simulink model "SVPWM2017a"  (R2017a)
settings: Solver=FixedStepAuto  StartTime=0.0  StopTime=0.1  RelTol=1e-3
values from neighbouring files (symbols this model uses):
  pxyz = sqrt(3) *Tsw / Vdc    [setting.m]
  Tsw = 1 / fsw    (= 0.0001)    [setting.m]
  Vdc = 500    [setting.m]
libraries: powerlib x11, simulink x4, powerlib_meascontrol x1
settings Model: Creator=d  LastModifiedBy=d
settings DataIOCC: ReturnWorkspaceOutputs=on
settings DebuggingCC: UnconnectedInputMsg=none  UnconnectedOutputMsg=none  UnconnectedLineMsg=none
settings ModelReferenceCC: EnableRefExpFcnMdlSchedulingChecks=off
settings SFSimCC: SimUseLocalCustomCode=on
settings RTWCC: RTWUseLocalCustomCode=on

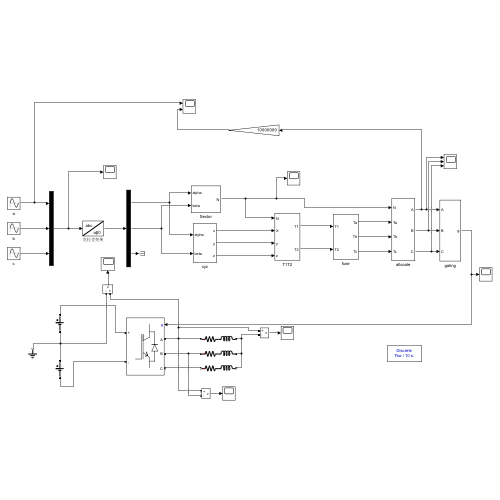
[thumbnail: Simulink's stored preview of the top-level diagram]
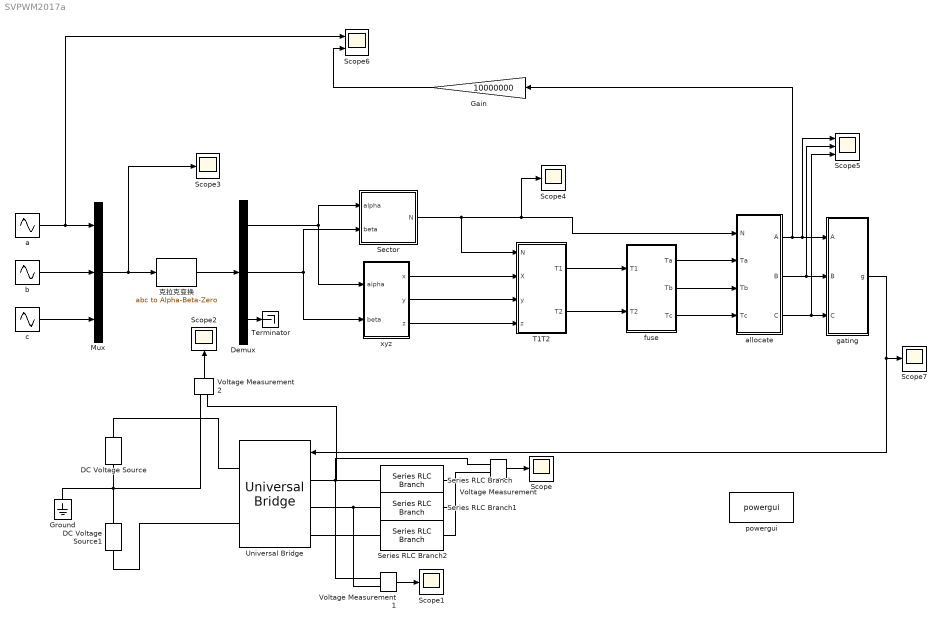
== system SVPWM2017a ==
  DC Voltage Source : powerlib/Electrical Sources/DC Voltage Source  Amplitude=Vdc / 2  Measurements=None
  DC Voltage Source1 : powerlib/Electrical Sources/DC Voltage Source  Amplitude=Vdc / 2  Measurements=None
  Demux : Demux  Outputs=3
  Gain : Gain  Gain=10000000
  Ground : powerlib/Elements/Ground  LConnTagsString=a
  Mux : Mux  Inputs=3
  Scope{,1..4,7} (6 alike) : Scope
  Scope5 : Scope  NumInputPorts=3
  Scope6 : Scope  NumInputPorts=2
  Sector : Subsystem
  Series RLC Branch : powerlib/Elements/Series RLC Branch  LConnTagsString=__new0  RConnTagsString=__new0  BranchType=RL  Resistance=1  Inductance=1e-3  SetiL0=off  InitialCurrent=0  Capacitance=1e-6  Setx0=off  InitialVoltage=0  Measurements=None
  Series RLC Branch1 : powerlib/Elements/Series RLC Branch  LConnTagsString=__new0  RConnTagsString=__new0  BranchType=RL  Resistance=1  Inductance=1e-3  SetiL0=off  InitialCurrent=0  Capacitance=1e-6  Setx0=off  InitialVoltage=0  Measurements=None
  Series RLC Branch2 : powerlib/Elements/Series RLC Branch  LConnTagsString=__new0  RConnTagsString=__new0  BranchType=RL  Resistance=1  Inductance=1e-3  SetiL0=off  InitialCurrent=0  Capacitance=1e-6  Setx0=off  InitialVoltage=0  Measurements=None
  T1T2 : Subsystem
  Terminator : Terminator
  Universal Bridge : powerlib/Power Electronics/Universal Bridge  Arms=3  SnubberResistance=1e5  SnubberCapacitance=inf  Device=IGBT / Diodes  Ron=1e-3  Lon=0  ForwardVoltages="[  0  0  ]"  ForwardVoltage=0  GTOparameters=[ 10e-6 , 20e-6 ]  IGBTparameters=[ 1e-6 , 2e-6 ]  Measurements=None  Measurements_2=None  converterType=Rectifier
  Voltage Measurement : powerlib/Measurements/Voltage Measurement  PhasorSimulation=off  OutputType=Complex  PSBequivalent=0
  Voltage Measurement1 : powerlib/Measurements/Voltage Measurement  PhasorSimulation=off  OutputType=Complex  PSBequivalent=0
  Voltage Measurement2 : powerlib/Measurements/Voltage Measurement  PhasorSimulation=off  OutputType=Complex  PSBequivalent=0
  a : Sin  Amplitude=(220 * sqrt(2)) / sqrt(3)  Frequency=50*2*pi  SampleTime=0
  allocate : Subsystem
  b : Sin  Amplitude=(220 * sqrt(2)) / sqrt(3)  Frequency=50*2*pi  Phase=-pi*2/3  SampleTime=0
  c : Sin  Amplitude=(220 * sqrt(2)) / sqrt(3)  Frequency=50*2*pi  Phase=-pi*4/3  SampleTime=0
  fuse : Subsystem
  gating : Subsystem
  powergui : powerlib/powergui  Priority=1  SimulationMode=Discrete  SampleTime=Tsw / 10  frequency=60  Iterations=50  frequencyindice=0  Pbase=100e6  ErrMax=1e-4  UnitsV=kV  UnitsW=MW  buscounter=0  FunctionMessages=off  echomessages=off  EnableUseOfTLC=off  CurrentSourceSwitches=off  DisableSnubberDevices=off  DisableRonSwitches=off  DisableVfSwitches=off  DisplayEquations=off  AutomaticDiscreteSolvers=off  SolverType=Tustin/Backward Euler (TBE)  Interpol=off  ExternalGateDelay=off  methode=off  Ts=100  x0status=blocks  SPID=on  SwTol=0  HookPort=off  NonlinearTolerance=1e-4  nMaxIteration=100  ContinueOnMaxIteration=off  RestoreLinks=warning  ResistiveCurrentMeasurement=off  Frange=[0:2:500]  Ylog=off  Xlog=on  ShowGrid=off  save=off  variable=ZData  structure=0  ZoomFFT=off  StartTime=0.0  cycles=1  DisplayStyle=1  fundamental=60  FreqAxis=off  MaxFrequency=1000  frequencyindicesteady=1  RmsSteady=1  display=off
  xyz : Subsystem
  克拉克变换 : powerlib_meascontrol/Transformations/abc to Alpha-Beta-Zero
  wires:
  Sector/1(N) -> T1T2/1(N), Scope4/1, allocate/1(N)
  xyz/1(x) -> T1T2/2(X)
  xyz/2(y) -> T1T2/3(y)
  xyz/3(z) -> T1T2/4(z)
  T1T2/1(T1) -> fuse/1(T1)
  T1T2/2(T2) -> fuse/2(T2)
  fuse/1(Ta) -> allocate/2(Ta)
  fuse/2(Tb) -> allocate/3(Tb)
  fuse/3(Tc) -> allocate/4(Tc)
  allocate/1(A) -> Gain/1, Scope5/1, gating/1(A)
  allocate/2(B) -> Scope5/2, gating/2(B)
  allocate/3(C) -> Scope5/3, gating/3(C)
  a/1 -> Scope6/1, Mux/1
  b/1 -> Mux/2
  c/1 -> Mux/3
  Mux/1 -> Scope3/1, 克拉克变换/1
  克拉克变换/1 -> Demux/1
  Demux/1 -> Sector/1(alpha), xyz/1(alpha)
  Demux/2 -> Sector/2(beta), xyz/2(beta)
  Demux/3 -> Terminator/1
  gating/1(g) -> Scope7/1, Universal Bridge/1
  Voltage Measurement/1 -> Scope/1
  Voltage Measurement1/1 -> Scope1/1
  Voltage Measurement2/1 -> Scope2/1
  Gain/1 -> Scope6/2
  connections:
  DC Voltage Source1/RConn1 -- Voltage Measurement2/LConn2 -- Ground/LConn1 -- DC Voltage Source/LConn1
  DC Voltage Source/RConn1 -- Universal Bridge/RConn1
  DC Voltage Source1/LConn1 -- Universal Bridge/RConn2
  Universal Bridge/LConn1 -- Voltage Measurement2/LConn1 -- Voltage Measurement/LConn1 -- Voltage Measurement1/LConn1 -- Series RLC Branch/LConn1
  Universal Bridge/LConn2 -- Voltage Measurement1/LConn2 -- Series RLC Branch1/LConn1
  Universal Bridge/LConn3 -- Series RLC Branch2/LConn1
  Series RLC Branch/RConn1 -- Voltage Measurement/LConn2 -- Series RLC Branch1/RConn1 -- Series RLC Branch2/RConn1

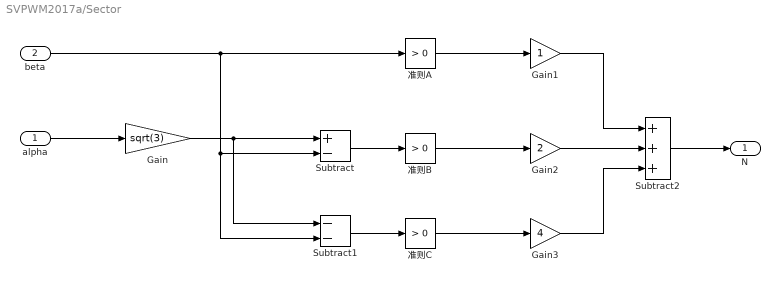
== system SVPWM2017a/Sector ==
  alpha : Inport
  beta : Inport  Port=2
  Gain : Gain  Gain=sqrt(3)
  Gain1 : Gain
  Gain2 : Gain  Gain=2
  Gain3 : Gain  Gain=4
  Subtract : Sum  Inputs=+-
  Subtract1 : Sum  Inputs=--
  Subtract2 : Sum  Inputs=+++
  准则A : simulink/Logic and Bit Operations/Compare To Constant  relop=>  const=0  OutDataTypeStr=boolean
  准则B : simulink/Logic and Bit Operations/Compare To Constant  relop=>  const=0  OutDataTypeStr=boolean
  准则C : simulink/Logic and Bit Operations/Compare To Constant  relop=>  const=0  OutDataTypeStr=boolean
  N : Outport
  wires:
  beta/1 -> Subtract1/2, Subtract/2, 准则A/1
  alpha/1 -> Gain/1
  Gain/1 -> Subtract1/1, Subtract/1
  Subtract/1 -> 准则B/1
  Subtract1/1 -> 准则C/1
  准则C/1 -> Gain3/1
  准则B/1 -> Gain2/1
  准则A/1 -> Gain1/1
  Gain1/1 -> Subtract2/1
  Gain2/1 -> Subtract2/2
  Gain3/1 -> Subtract2/3
  Subtract2/1 -> N/1

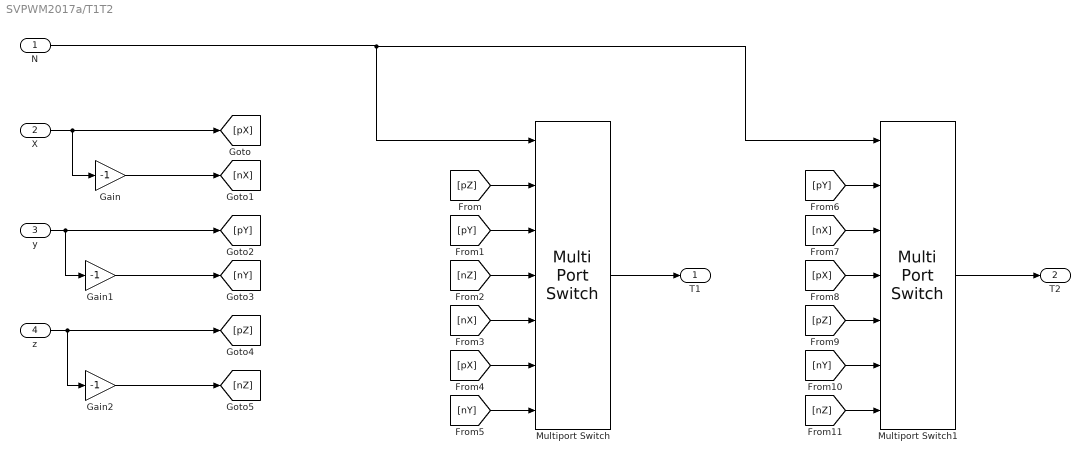
== system SVPWM2017a/T1T2 ==
  N : Inport
  X : Inport  Port=2
  y : Inport  Port=3
  z : Inport  Port=4
  Gain : Gain  Gain=-1
  Gain1 : Gain  Gain=-1
  Gain2 : Gain  Gain=-1
  Multiport Switch : MultiPortSwitch  Inputs=6
  Multiport Switch1 : MultiPortSwitch  Inputs=6
  T1 : Outport
  T2 : Outport  Port=2
  wires:
  X/1 -> [pX], Gain/1
  y/1 -> [pY], Gain1/1
  z/1 -> Gain2/1, [pZ]
  Gain/1 -> [nX]
  Gain1/1 -> [nY]
  Gain2/1 -> [nZ]
  Multiport Switch/1 -> T1/1
  Multiport Switch1/1 -> T2/1
  N/1 -> Multiport Switch1/1, Multiport Switch/1
  [pZ] -> Multiport Switch/2
  [pY] -> Multiport Switch/3
  [nZ] -> Multiport Switch/4
  [nX] -> Multiport Switch/5
  [pX] -> Multiport Switch/6
  [nY] -> Multiport Switch/7
  [pY] -> Multiport Switch1/2
  [nX] -> Multiport Switch1/3
  [pX] -> Multiport Switch1/4
  [pZ] -> Multiport Switch1/5
  [nY] -> Multiport Switch1/6
  [nZ] -> Multiport Switch1/7

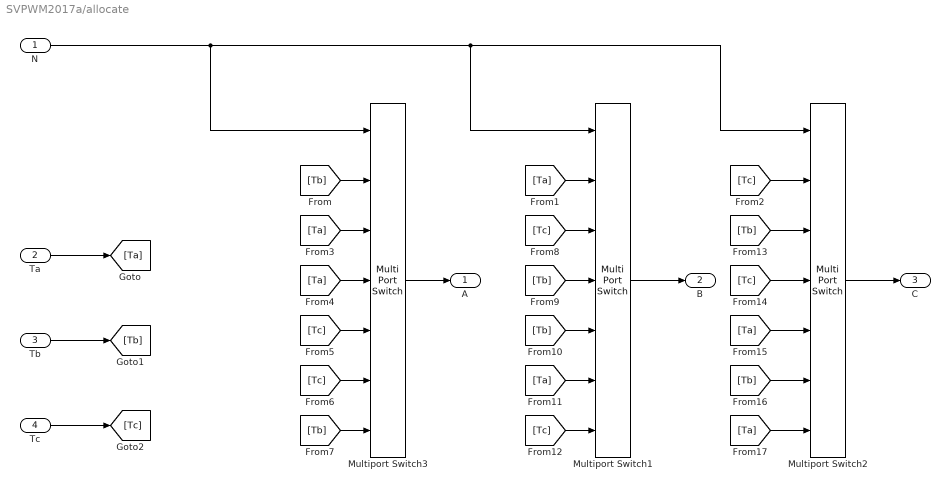
== system SVPWM2017a/allocate ==
  N : Inport
  Ta : Inport  Port=2
  Tb : Inport  Port=3
  Tc : Inport  Port=4
  Multiport Switch1 : MultiPortSwitch  Inputs=6
  Multiport Switch2 : MultiPortSwitch  Inputs=6
  Multiport Switch3 : MultiPortSwitch  Inputs=6
  A : Outport
  B : Outport  Port=2
  C : Outport  Port=3
  wires:
  Tc/1 -> [Tc]
  Tb/1 -> [Tb]
  Ta/1 -> [Ta]
  Multiport Switch2/1 -> C/1
  Multiport Switch3/1 -> A/1
  Multiport Switch1/1 -> B/1
  N/1 -> Multiport Switch3/1, Multiport Switch1/1, Multiport Switch2/1
  [Tb] -> Multiport Switch3/2
  [Ta] -> Multiport Switch1/2
  [Tc] -> Multiport Switch2/2
  [Ta] -> Multiport Switch3/3
  [Ta] -> Multiport Switch3/4
  [Tc] -> Multiport Switch3/5
  [Tc] -> Multiport Switch3/6
  [Tb] -> Multiport Switch3/7
  [Tc] -> Multiport Switch1/3
  [Tb] -> Multiport Switch1/4
  [Tb] -> Multiport Switch1/5
  [Ta] -> Multiport Switch1/6
  [Tc] -> Multiport Switch1/7
  [Tb] -> Multiport Switch2/3
  [Tc] -> Multiport Switch2/4
  [Ta] -> Multiport Switch2/5
  [Tb] -> Multiport Switch2/6
  [Ta] -> Multiport Switch2/7

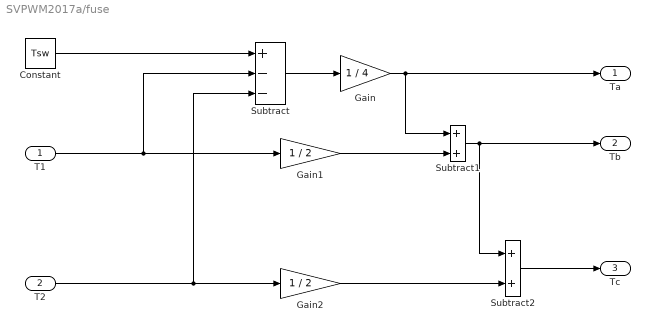
== system SVPWM2017a/fuse ==
  T1 : Inport
  T2 : Inport  Port=2
  Constant : Constant  Value=Tsw
  Gain : Gain  Gain=1 / 4
  Gain1 : Gain  Gain=1 / 2
  Gain2 : Gain  Gain=1 / 2
  Subtract : Sum  Inputs=+--
  Subtract1 : Sum
  Subtract2 : Sum
  Ta : Outport
  Tb : Outport  Port=2
  Tc : Outport  Port=3
  wires:
  Constant/1 -> Subtract/1
  T1/1 -> Gain1/1, Subtract/2
  T2/1 -> Gain2/1, Subtract/3
  Subtract/1 -> Gain/1
  Gain/1 -> Subtract1/1, Ta/1
  Gain1/1 -> Subtract1/2
  Subtract1/1 -> Subtract2/1, Tb/1
  Subtract2/1 -> Tc/1
  Gain2/1 -> Subtract2/2

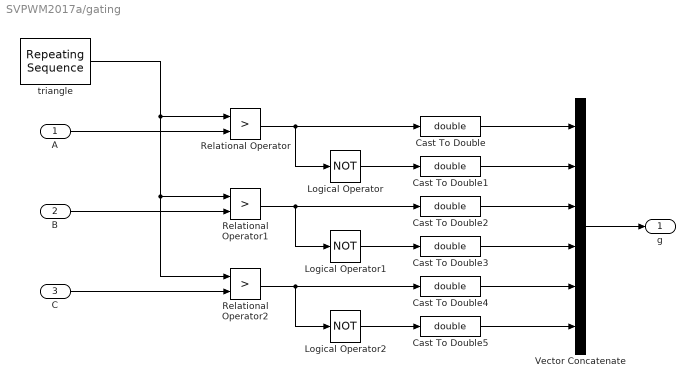
== system SVPWM2017a/gating ==
  A : Inport
  B : Inport  Port=2
  C : Inport  Port=3
  Cast To Double{,1..5} (6 alike) : DataTypeConversion  OutDataTypeStr=double
  Logical Operator : Logic  Operator=NOT  AllPortsSameDT=off  OutDataTypeStr=boolean
  Logical Operator1 : Logic  Operator=NOT  AllPortsSameDT=off  OutDataTypeStr=boolean
  Logical Operator2 : Logic  Operator=NOT  AllPortsSameDT=off  OutDataTypeStr=boolean
  Relational Operator : RelationalOperator  Operator=>  OutDataTypeStr=boolean  RndMeth=Simplest
  Relational Operator1 : RelationalOperator  Operator=>  OutDataTypeStr=boolean  RndMeth=Simplest
  Relational Operator2 : RelationalOperator  Operator=>  OutDataTypeStr=boolean  RndMeth=Simplest
  Vector Concatenate : Concatenate  NumInputs=6
  triangle : simulink/Sources/Repeating Sequence  rep_seq_t=[0 Tsw/2 Tsw]  rep_seq_y=[0 Tsw/2 0]
  g : Outport
  wires:
  triangle/1 -> Relational Operator/1, Relational Operator2/1, Relational Operator1/1
  A/1 -> Relational Operator/2
  B/1 -> Relational Operator1/2
  C/1 -> Relational Operator2/2
  Relational Operator1/1 -> Cast To Double2/1, Logical Operator1/1
  Relational Operator/1 -> Cast To Double/1, Logical Operator/1
  Relational Operator2/1 -> Cast To Double4/1, Logical Operator2/1
  Logical Operator/1 -> Cast To Double1/1
  Logical Operator1/1 -> Cast To Double3/1
  Logical Operator2/1 -> Cast To Double5/1
  Cast To Double/1 -> Vector Concatenate/1
  Cast To Double1/1 -> Vector Concatenate/2
  Cast To Double2/1 -> Vector Concatenate/3
  Cast To Double3/1 -> Vector Concatenate/4
  Cast To Double4/1 -> Vector Concatenate/5
  Cast To Double5/1 -> Vector Concatenate/6
  Vector Concatenate/1 -> g/1

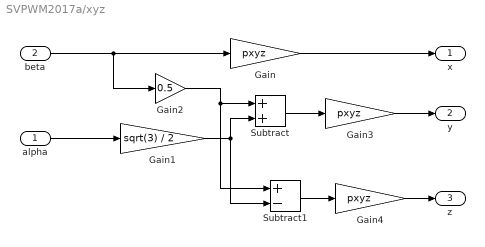
== system SVPWM2017a/xyz ==
  alpha : Inport
  beta : Inport  Port=2
  Gain : Gain  Gain=pxyz
  Gain1 : Gain  Gain=sqrt(3) / 2
  Gain2 : Gain  Gain=0.5
  Gain3 : Gain  Gain=pxyz
  Gain4 : Gain  Gain=pxyz
  Subtract : Sum
  Subtract1 : Sum  Inputs=+-
  x : Outport
  y : Outport  Port=2
  z : Outport  Port=3
  wires:
  beta/1 -> Gain2/1, Gain/1
  Gain/1 -> x/1
  alpha/1 -> Gain1/1
  Gain2/1 -> Subtract1/1, Subtract/1
  Gain1/1 -> Subtract/2, Subtract1/2
  Gain3/1 -> y/1
  Subtract/1 -> Gain3/1
  Gain4/1 -> z/1
  Subtract1/1 -> Gain4/1
